simulink model "EngineCtrl_V1"  (R2018a)
settings: Solver=VariableStepAuto  StartTime=0.0  StopTime=10.0  FixedStep=sampletime  RelTol=1e-3  EnableMultiTasking=on
PreLoadFcn:
  | EngineCtrl_V1_BusInfo
libraries: simulink x2
settings Model: Creator=IAEC nishito  LastModifiedBy=nishito
settings DataIOCC: LimitDataPoints=on  SaveFormat=Array  SignalLoggingSaveFormat=ModelDataLogs  SaveOutput=off  SaveTime=off
settings OptimizationCC: DefaultParameterBehavior=Inlined  ExpressionDepthLimit=2147483647  LifeSpan=inf
settings DebuggingCC: SolverPrmCheckMsg=warning  FcnCallInpInsideContextMsg=warning  StateNameClashWarn=warning  SFUnexpectedBacktrackingDiag=warning  SFNoUnconditionalDefaultTransitionDiag=warning  SFExecutionAtInitializationDiag=none
settings HardwareCC: ProdBitPerPointer=32  ProdBitPerSizeT=32  ProdBitPerPtrDiffT=32  ProdLargestAtomicFloat=None  ProdIntDivRoundTo=Undefined  ProdEndianess=Unspecified  ProdWordSize=32  ProdHWDeviceType=32-bit Generic
settings ModelReferenceCC: UpdateModelReferenceTargets=IfOutOfDate  PropagateSignalLabelsOutOfModel=off
settings CodeAppCC: StateflowObjectComments=on
settings GRTTargetCC: TargetLangStandard=C89/C90 (ANSI)  GeneratePreprocessorConditionals=Disable all  CombineOutputUpdateFcns=off  GRTInterface=on
settings ConfigComp: CovMetricSettings=dw  CovHtmlReporting=on  CovSaveCumulativeToWorkspaceVar=on  CovSaveSingleToWorkspaceVar=on  CovExternalEMLEnable=off

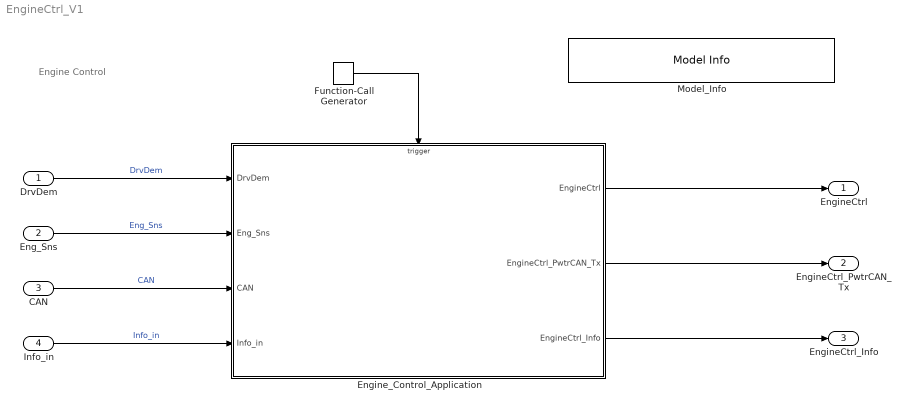
== system EngineCtrl_V1 ==
  note: Engine Control
  DrvDem : Inport  OutDataTypeStr=Bus: Driver_demand_Bus
      settings: AttributesFormatString=%<OutDataTypeStr>
  Eng_Sns : Inport  Port=2  OutDataTypeStr=Bus: Engine_sensor_Bus
      settings: AttributesFormatString=%<OutDataTypeStr>
  CAN : Inport  Port=3  OutDataTypeStr=Bus: CAN_Bus
      settings: AttributesFormatString=<%<OutDataTypeStr>>
  Info_in : Inport  Port=4  OutDataTypeStr=Bus: EngineCtrl_Info_in_Bus
      settings: AttributesFormatString=%<OutDataTypeStr>
  Engine_Control_Application : Subsystem
  Function-Call Generator : simulink/Ports & Subsystems/Function-Call Generator  sample_time=0.01  numberOfIterations=1
      settings: AttributesFormatString=<sample_time=%<sample_time>>
  Model_Info : simulink/Model-Wide Utilities/Model Info  Frame=on  DisplayStringWithTags=|  HorizontalTextAlignment=Left  LeftAlignmentValue=0.02
      | Version  %<ModelVersion>
      | LastModifided by %<LastModifiedBy>  Date %<LastModificationDate>
      | Description  %<Description>
  EngineCtrl : Outport  OutDataTypeStr=Bus: EngineCtrl_Bus
      settings: AttributesFormatString=<%<OutDataTypeStr>>
  EngineCtrl_PwtrCAN_Tx : Outport  Port=2  OutDataTypeStr=Bus: EngineCtrl_PwtrCAN_Tx_Bus
      settings: AttributesFormatString=<%<OutDataTypeStr>>
  EngineCtrl_Info : Outport  Port=3  OutDataTypeStr=Bus: EngineCtrl_Info_Bus
      settings: AttributesFormatString=<%<OutDataTypeStr>>
  wires:
  CAN/1 -> Engine_Control_Application/3(CAN)  "CAN"
  DrvDem/1 -> Engine_Control_Application/1(DrvDem)  "DrvDem"
  Eng_Sns/1 -> Engine_Control_Application/2(Eng_Sns)  "Eng_Sns"
  Function-Call Generator/1 -> Engine_Control_Application/Trigger
  Engine_Control_Application/2(EngineCtrl_PwtrCAN_Tx) -> EngineCtrl_PwtrCAN_Tx/1
  Engine_Control_Application/1(EngineCtrl) -> EngineCtrl/1
  Engine_Control_Application/3(EngineCtrl_Info) -> EngineCtrl_Info/1
  Info_in/1 -> Engine_Control_Application/4(Info_in)  "Info_in"

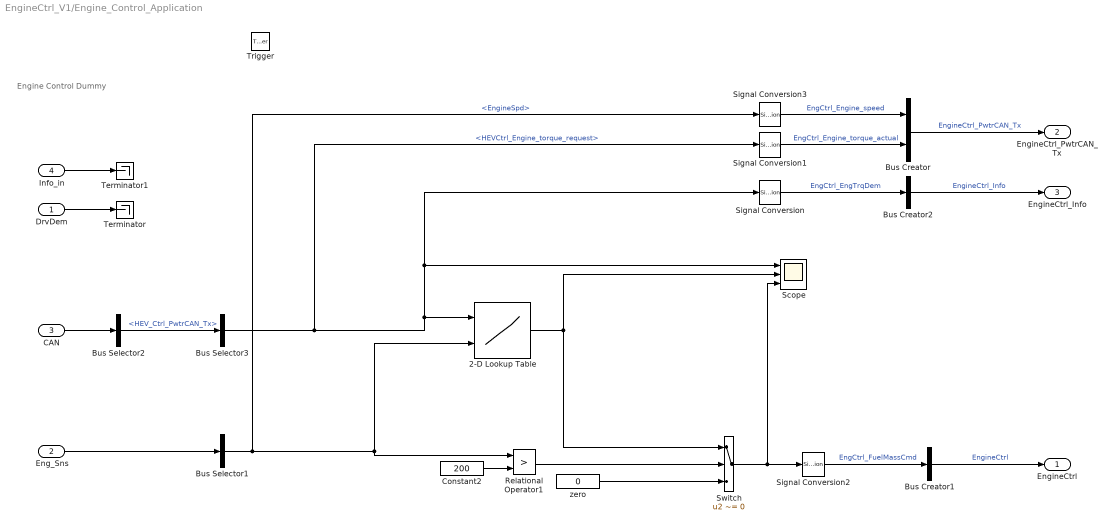
== system EngineCtrl_V1/Engine_Control_Application ==
  note: Engine Control Dummy
  DrvDem : Inport
  Eng_Sns : Inport  Port=2
  CAN : Inport  Port=3
  Info_in : Inport  Port=4
  Trigger : TriggerPort  TriggerType=function-call  VariantControl=Variant  PortDimensions=1
  2-D Lookup Table : Lookup_n-D  BreakpointsForDimension1=[0 400]  BreakpointsForDimension2=[0 200 600 1000]  Table=[0 10 0 0; 70 70 70 70]  InternalRulePriority=Speed  RndMeth=Simplest  InputSameDT=on
  Bus Creator : BusCreator  Inputs=2  OutDataTypeStr=Bus: EngineCtrl_PwtrCAN_Tx_Bus
      settings: AttributesFormatString=%<OutDataTypeStr>
  Bus Creator1 : BusCreator  Inputs=1  OutDataTypeStr=Bus: EngineCtrl_Bus
      settings: AttributesFormatString=%<OutDataTypeStr>
  Bus Creator2 : BusCreator  Inputs=1  OutDataTypeStr=Bus: EngineCtrl_Info_Bus
      settings: AttributesFormatString=%<OutDataTypeStr>
  Bus Selector1 : BusSelector  OutputSignals=EngineSpd
  Bus Selector2 : BusSelector  OutputSignals=PwtrCAN.HEV_Ctrl_PwtrCAN_Tx
  Bus Selector3 : BusSelector  OutputSignals=HEVCtrl_Engine_torque_request
  Constant2 : Constant  Value=200
  Relational Operator1 : RelationalOperator  Operator=>  OutDataTypeStr=boolean  RndMeth=Nearest
  Scope : Scope  NumInputPorts=3
  Signal Conversion{,1..3} (4 alike) : SignalConversion  OverrideOpt=off
  Switch : Switch  Criteria=u2 ~= 0  Threshold=0.5  SaturateOnIntegerOverflow=on
      settings: AttributesFormatString=<%<Criteria>>
  Terminator : Terminator
  Terminator1 : Terminator
  zero : Constant  Value=0
  EngineCtrl : Outport
  EngineCtrl_PwtrCAN_Tx : Outport  Port=2
  EngineCtrl_Info : Outport  Port=3
  wires:
  DrvDem/1 -> Terminator/1
  CAN/1 -> Bus Selector2/1
  Eng_Sns/1 -> Bus Selector1/1
  Bus Creator/1 -> EngineCtrl_PwtrCAN_Tx/1  "EngineCtrl_PwtrCAN_Tx"
  Bus Creator1/1 -> EngineCtrl/1  "EngineCtrl"
  Bus Creator2/1 -> EngineCtrl_Info/1  "EngineCtrl_Info"
  2-D Lookup Table/1 -> Switch/1, Scope/2
  Switch/1 -> Scope/3, Signal Conversion2/1
  zero/1 -> Switch/3
  Signal Conversion/1 -> Bus Creator2/1  "EngCtrl_EngTrqDem"
  Signal Conversion1/1 -> Bus Creator/2  "EngCtrl_Engine_torque_actual"
  Signal Conversion2/1 -> Bus Creator1/1  "EngCtrl_FuelMassCmd"
  Constant2/1 -> Relational Operator1/2
  Relational Operator1/1 -> Switch/2
  Bus Selector2/1 -> Bus Selector3/1  "<HEV_Ctrl_PwtrCAN_Tx>"
  Bus Selector1/1 -> Signal Conversion3/1, 2-D Lookup Table/2, Relational Operator1/1  "<EngineSpd>"
  Bus Selector3/1 -> Signal Conversion1/1, 2-D Lookup Table/1, Signal Conversion/1, Scope/1  "<HEVCtrl_Engine_torque_request>"
  Signal Conversion3/1 -> Bus Creator/1  "EngCtrl_Engine_speed"
  Info_in/1 -> Terminator1/1
